simulink model "app_Main100msMgr"  (R2019b)
settings: Solver=FixedStepDiscrete  StartTime=0.0  StopTime=10.0  FixedStep=0.1  RelTol=1e-3  EnableMultiTasking=on
PreLoadFcn:
  | try
  |    tapas_types('load');
  | catch
  |   disp('TAPAS WARNING: Tapas Types could not be loaded ...');
  | end
  | 
  | try
  |   app_types('load');
  | catch
  |   currdir =pwd;
  |   try
  |     cd('..\app_types\');
  |     app_types('load');
  |     cd(currdir);
  |   catch
  |     try
  |        cd('..\..\app_types\');
  |        app_types('load');
  |        cd(currdir);
  |     catch
  |        cd(currdir);
  |        disp('TAPAS WARNING: Application Types could not be loaded ...');
  |     end
  |   end
  |   try
  |       clear currdir;
  |   catch
  |      %Do nothing
  |   end
  | end
settings Model: Creator=kmansour  LastModifiedBy=depl_
settings DataIOCC: LimitDataPoints=on  SaveFormat=Array  ReturnWorkspaceOutputs=off
settings OptimizationCC: LifeSpan=1  EfficientTunableParamExpr=on
settings DebuggingCC: AllowSymbolicDim=off  SFUnexpectedBacktrackingDiag=warning  SFNoUnconditionalDefaultTransitionDiag=warning  SFExecutionAtInitializationDiag=none  ArithmeticOperatorsInVariantConditions=warning
settings HardwareCC: ProdBitPerPointer=32  ProdBitPerSizeT=32  ProdBitPerPtrDiffT=32  ProdLargestAtomicInteger=Long  ProdLargestAtomicFloat=Double  ProdEndianess=BigEndian  ProdWordSize=32  ProdHWDeviceType=Texas Instruments->TMS570 Cortex-R4
settings ModelReferenceCC: ModelReferenceNumInstancesAllowed=Single  PropagateSignalLabelsOutOfModel=off
settings SFSimCC: SimUseLocalCustomCode=off  MATLABDynamicMemAlloc=off  CustomCodeUndefinedFunction=UseInterfaceOnly
settings RTWCC: SystemTargetFile=ert.tlc  GenCodeOnly=on  TemplateMakefile=ert_default_tmf  GenerateReport=on  RTWUseLocalCustomCode=off  IncludeHyperlinkInReport=on  LaunchReport=on  GenerateTraceInfo=on  GenerateTraceReport=on  GenerateTraceReportSl=on  GenerateTraceReportSf=on  GenerateTraceReportEml=on
settings CodeAppCC: IgnoreCustomStorageClasses=off  MaxIdLength=63  StateflowObjectComments=on
settings ERTTargetCC: MultiwordLength=2048  GenerateSampleERTMain=on  GenerateASAP2=on  RTWCAPISignals=on  RTWCAPIParams=on  RTWCAPIStates=on  RTWCAPIRootIO=on  ERTSrcFileBannerTemplate=deMCD_code_template.cgt  ERTHdrFileBannerTemplate=deMCD_code_template.cgt  ERTDataSrcFileTemplate=deMCD_code_template.cgt  ERTDataHdrFileTemplate=deMCD_code_template.cgt  ERTCustomFileTemplate=example_file_process.tlc  ConvertIfToSwitch=off  SuppressUnreachableDefaultCases=off
settings ConfigComp: CovMetricSettings=dw  CovHtmlReporting=on  CovSaveCumulativeToWorkspaceVar=on  CovSaveSingleToWorkspaceVar=on  CovExternalEMLEnable=off

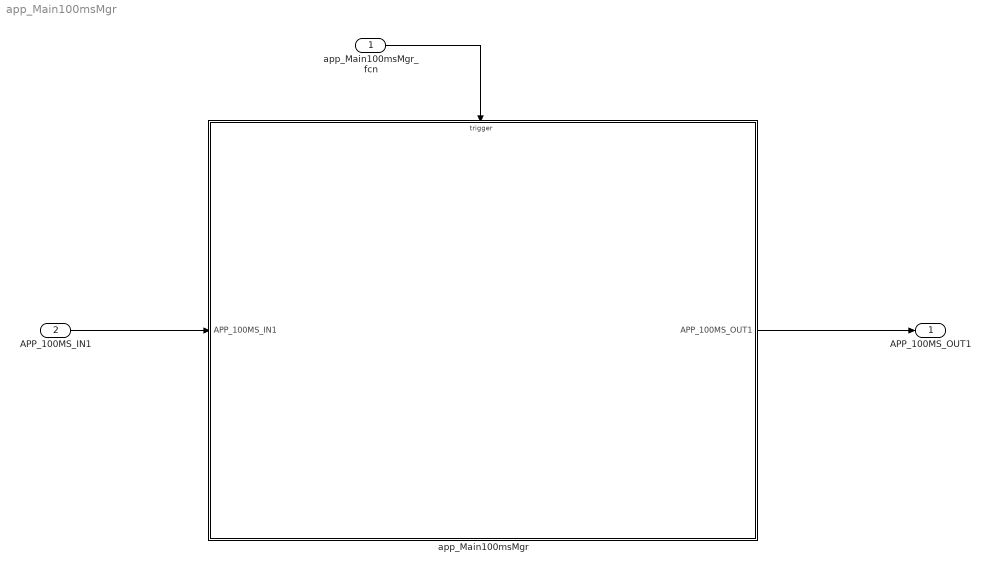
== system app_Main100msMgr ==
  app_Main100msMgr_fcn : Inport  SampleTime=100e-3  OutputFunctionCall=on
  APP_100MS_IN1 : Inport  Port=2
  app_Main100msMgr : Subsystem
      mask Display: image(('Devise Logo.JPG'),'center');
  APP_100MS_OUT1 : Outport
  wires:
  app_Main100msMgr_fcn/1 -> app_Main100msMgr/Trigger
  APP_100MS_IN1/1 -> app_Main100msMgr/1(APP_100MS_IN1)
  app_Main100msMgr/1(APP_100MS_OUT1) -> APP_100MS_OUT1/1

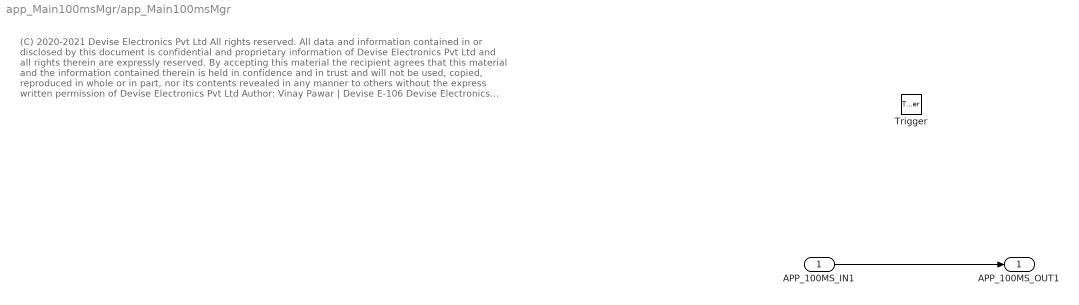
== system app_Main100msMgr/app_Main100msMgr ==
  note: (C) 2020-2021 Devise Electronics Pvt Ltd
      | All rights reserved.
      |
      | All data and information contained in or disclosed by this document is confidential and proprietary information of Devise Electronics Pvt Ltd and all rights therein are expressly reserved. By accepting this material the recipient agrees that this material and the information contained therein is held in confidence and in trust and will not be used, copied, reproduced in whole or in part, nor its contents revealed in any manner to others without the express written permission of Devise Electronics Pvt Ltd
      |
      | Author: Vinay Pawar | Devise E-106
      |
      | Devise Electronics Pvt Ltd
      | Pune,
      | India
      | E-mail: Shekhar.malani@deviseelectronics.com
  APP_100MS_IN1 : Inport
  Trigger : TriggerPort  TriggerType=function-call  VariantControl=Variant  SampleTimeType=periodic  SampleTime=-1  PortDimensions=1
  APP_100MS_OUT1 : Outport
  wires:
  APP_100MS_IN1/1 -> APP_100MS_OUT1/1
